simulink model "sim_Exp81_part2"  (R2019b)
settings: Solver=VariableStepAuto  StartTime=0.0  StopTime=10.0  RelTol=1e-3
undefined symbols (not defined in the file): GP_den, GP_num, Kp_part1
settings Model: Creator=sgxgong4  LastModifiedBy=xg
settings SFSimCC: CustomCodeUndefinedFunction=UseInterfaceOnly

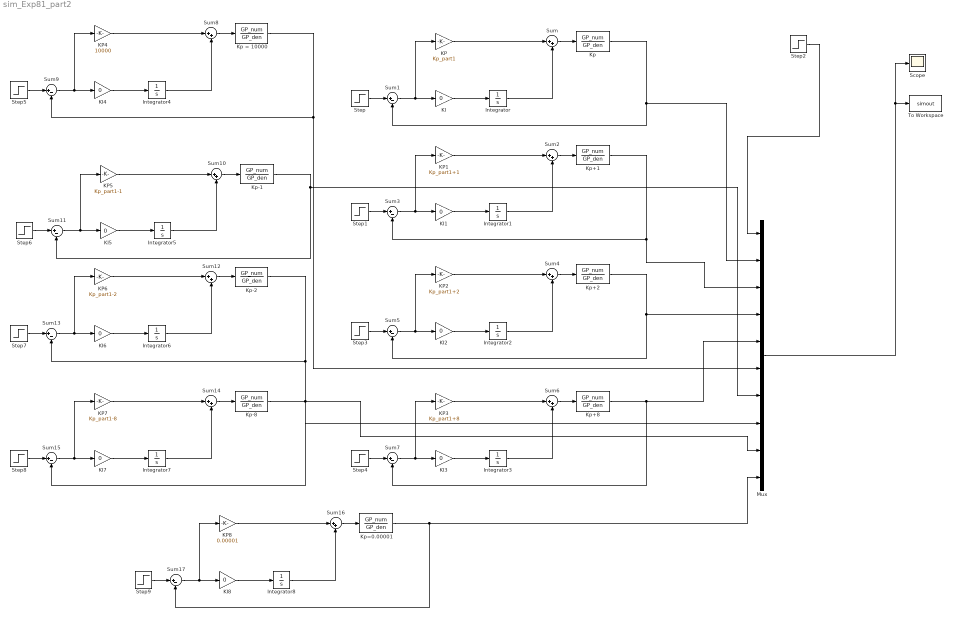
== system sim_Exp81_part2 ==
  Integrator{,1..8} (9 alike) : Integrator
  KI{,1..8} (9 alike) : Gain  Gain=0
  KP : Gain  Gain=Kp_part1
  KP1 : Gain  Gain=Kp_part1+1
  KP2 : Gain  Gain=Kp_part1+2
  KP3 : Gain  Gain=Kp_part1+8
  KP4 : Gain  Gain=10000
  KP5 : Gain  Gain=Kp_part1-1
  KP6 : Gain  Gain=Kp_part1-2
  KP7 : Gain  Gain=Kp_part1-8
  KP8 : Gain  Gain=0.00001
  Kp : TransferFcn  Numerator=GP_num  Denominator=GP_den
  Kp = 10000 : TransferFcn  Numerator=GP_num  Denominator=GP_den
  Kp+1 : TransferFcn  Numerator=GP_num  Denominator=GP_den
  Kp+2 : TransferFcn  Numerator=GP_num  Denominator=GP_den
  Kp+8 : TransferFcn  Numerator=GP_num  Denominator=GP_den
  Kp-1 : TransferFcn  Numerator=GP_num  Denominator=GP_den
  Kp-2 : TransferFcn  Numerator=GP_num  Denominator=GP_den
  Kp-8 : TransferFcn  Numerator=GP_num  Denominator=GP_den
  Kp=0.00001 : TransferFcn  Numerator=GP_num  Denominator=GP_den
  Mux : Mux  Inputs=10
  Scope : Scope
  Step{,1..9} (10 alike) : Step  Time=0  SampleTime=0
  Sum{,2,4,6,8,10,12,14,16} (9 alike) : Sum  Inputs=|++
  Sum{1,3,5,7,9,11,13,15,17} (9 alike) : Sum  Inputs=|+-
  To Workspace : ToWorkspace  VariableName=simout  SaveFormat=Structure With Time  SampleTime=-1
  wires:
  KI/1 -> Integrator/1
  KP/1 -> Sum/1
  Integrator/1 -> Sum/2
  Sum1/1 -> KP/1, KI/1
  Step/1 -> Sum1/1
  Sum/1 -> Kp/1
  Kp/1 -> Sum1/2, Mux/2
  Mux/1 -> To Workspace/1, Scope/1
  Step2/1 -> Mux/1
  Integrator1/1 -> Sum2/2
  Kp+1/1 -> Mux/3, Sum3/2
  Sum2/1 -> Kp+1/1
  Step1/1 -> Sum3/1
  Sum3/1 -> KP1/1, KI1/1
  KI1/1 -> Integrator1/1
  KP1/1 -> Sum2/1
  Integrator2/1 -> Sum4/2
  Kp+2/1 -> Sum5/2, Mux/4
  Sum4/1 -> Kp+2/1
  Step3/1 -> Sum5/1
  Sum5/1 -> KP2/1, KI2/1
  KI2/1 -> Integrator2/1
  KP2/1 -> Sum4/1
  Integrator3/1 -> Sum6/2
  Kp+8/1 -> Sum7/2, Mux/5
  Sum6/1 -> Kp+8/1
  Step4/1 -> Sum7/1
  Sum7/1 -> KP3/1, KI3/1
  KI3/1 -> Integrator3/1
  KP3/1 -> Sum6/1
  Integrator4/1 -> Sum8/2
  Kp = 10000/1 -> Sum9/2, Mux/6
  Sum8/1 -> Kp = 10000/1
  Step5/1 -> Sum9/1
  Sum9/1 -> KP4/1, KI4/1
  KI4/1 -> Integrator4/1
  KP4/1 -> Sum8/1
  Integrator5/1 -> Sum10/2
  Sum11/1 -> KP5/1, KI5/1
  Step6/1 -> Sum11/1
  Sum10/1 -> Kp-1/1
  KP5/1 -> Sum10/1
  KI5/1 -> Integrator5/1
  Kp-1/1 -> Mux/7, Sum11/2
  Integrator6/1 -> Sum12/2
  Sum13/1 -> KP6/1, KI6/1
  Step7/1 -> Sum13/1
  Sum12/1 -> Kp-2/1
  KP6/1 -> Sum12/1
  KI6/1 -> Integrator6/1
  Kp-2/1 -> Mux/8, Sum13/2
  Integrator7/1 -> Sum14/2
  Sum15/1 -> KP7/1, KI7/1
  Step8/1 -> Sum15/1
  Sum14/1 -> Kp-8/1
  KP7/1 -> Sum14/1
  KI7/1 -> Integrator7/1
  Kp-8/1 -> Mux/9, Sum15/2
  Integrator8/1 -> Sum16/2
  Sum17/1 -> KP8/1, KI8/1
  Step9/1 -> Sum17/1
  Sum16/1 -> Kp=0.00001/1
  KP8/1 -> Sum16/1
  KI8/1 -> Integrator8/1
  Kp=0.00001/1 -> Mux/10, Sum17/2
